simulink model "motor_position_control"  (Simulink 8.9)
settings: Solver=ode45  StartTime=0.0  StopTime=10.0  RelTol=1e-3  EnableMultiTasking=on
settings Model: SuppressorTable=22 serialization::archive 11 0 6 0 0 0 0 0  Creator=arturogilaparicio  LastModifiedBy=arturogilaparicio
settings DataIOCC: SignalLoggingSaveFormat=Dataset
settings DebuggingCC: UnderspecifiedInitializationDetection=Simplified  MergeDetectMultiDrivingBlocksExec=error  FcnCallInpInsideContextMsg=error  StateNameClashWarn=none
settings GRTTargetCC: CombineOutputUpdateFcns=on  GRTInterface=off

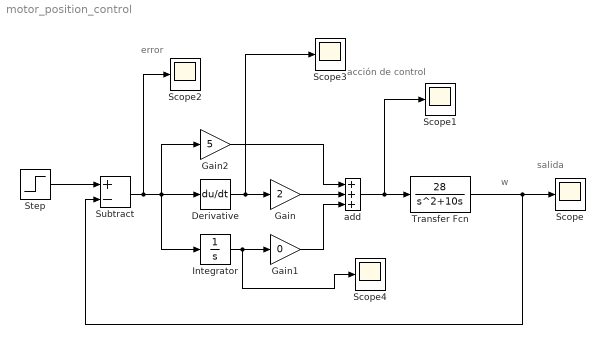
== system motor_position_control ==
  note: error
  note: acción de control
  note: salida
  note: w
  Derivative : Derivative
  Gain : Gain  Gain=2
  Gain1 : Gain  Gain=0
  Gain2 : Gain  Gain=5
  Integrator : Integrator
  Scope{,1..4} (5 alike) : Scope
  Step : Step  Time=0  After=5  SampleTime=0
  Subtract : Sum  Inputs=+-
  Transfer Fcn : TransferFcn  Numerator=[28]  Denominator=[1 10 0]
  add : Sum  Inputs=+++
  wires:
  add/1 -> Scope1/1, Transfer Fcn/1
  Gain/1 -> add/2
  Gain2/1 -> add/1
  Gain1/1 -> add/3
  Derivative/1 -> Scope3/1, Gain/1
  Integrator/1 -> Scope4/1, Gain1/1
  Subtract/1 -> Scope2/1, Integrator/1, Gain2/1, Derivative/1
  Step/1 -> Subtract/1
  Transfer Fcn/1 -> Scope/1, Subtract/2
